simulink model "rob_kuka_sim"  (R2018b)
settings: Solver=VariableStepAuto  StartTime=0.0  StopTime=90  RelTol=1e-3
values from neighbouring files (symbols this model uses):
  L_SB = 14.173    [rob_kuka.m]    (also in rob_kuka_pose.m)
  T = [T; 0,0,0,1]    [forKine.m]    (also in rob_kuka.m = zeros(n*4,4); rob_kuka_pose.m = zeros(n*4,4))
libraries: vrlib x17, dspmtrx3 x4
settings Model: Creator=szhao3  LastModifiedBy=szhao3
settings SFSimCC: SimUseLocalCustomCode=off
settings RTWCC: RTWUseLocalCustomCode=off

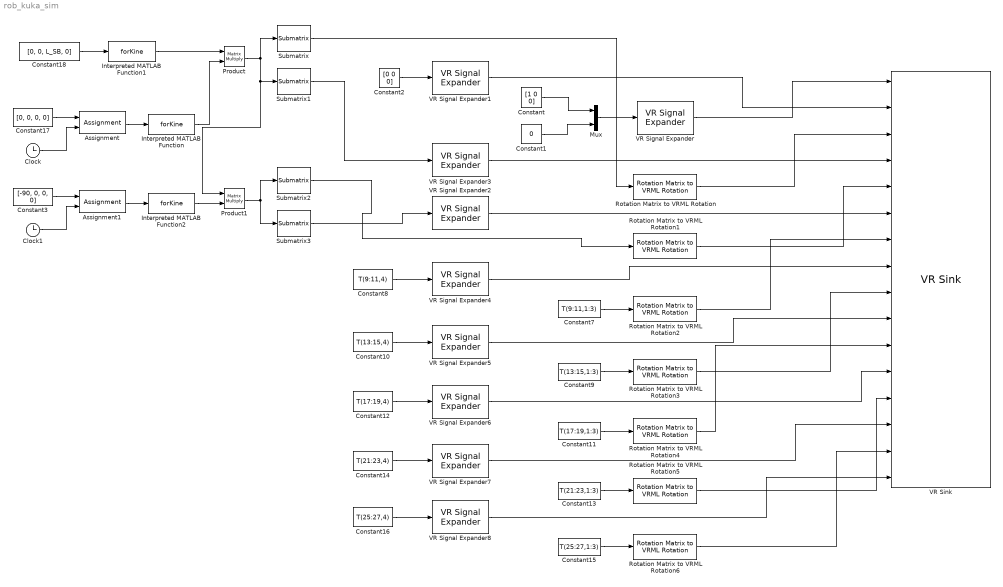
== system rob_kuka_sim ==
  Assignment : Assignment  DiagnosticForDimensions=Warning  IndexOptions=Index vector (dialog)  Indices=4  OutputSizes=1
  Assignment1 : Assignment  DiagnosticForDimensions=Warning  IndexOptions=Index vector (dialog)  Indices=4  OutputSizes=1
  Clock : Clock
  Clock1 : Clock
  Constant : Constant  Value=[1 0 0]  VectorParams1D=off
  Constant1 : Constant  Value=0
  Constant10 : Constant  Value=T(13:15,4)  VectorParams1D=off
  Constant11 : Constant  Value=T(17:19,1:3)  VectorParams1D=off
  Constant12 : Constant  Value=T(17:19,4)  VectorParams1D=off
  Constant13 : Constant  Value=T(21:23,1:3)  VectorParams1D=off
  Constant14 : Constant  Value=T(21:23,4)  VectorParams1D=off
  Constant15 : Constant  Value=T(25:27,1:3)  VectorParams1D=off
  Constant16 : Constant  Value=T(25:27,4)  VectorParams1D=off
  Constant17 : Constant  Value=[0, 0, 0, 0]  VectorParams1D=off
  Constant18 : Constant  Value=[0, 0, L_SB, 0]  VectorParams1D=off
  Constant2 : Constant  Value=[0 0 0]  VectorParams1D=off
  Constant3 : Constant  Value=[-90, 0, 0, 0]  VectorParams1D=off
  Constant7 : Constant  Value=T(9:11,1:3)  VectorParams1D=off
  Constant8 : Constant  Value=T(9:11,4)  VectorParams1D=off
  Constant9 : Constant  Value=T(13:15,1:3)  VectorParams1D=off
  Interpreted MATLAB Function : MATLABFcn  MATLABFcn=forKine  Output1D=off
  Interpreted MATLAB Function1 : MATLABFcn  MATLABFcn=forKine  Output1D=off
  Interpreted MATLAB Function2 : MATLABFcn  MATLABFcn=forKine  Output1D=off
  Mux : Mux  Inputs=2
  Product : Product  Multiplication=Matrix(*)
  Product1 : Product  Multiplication=Matrix(*)
  Rotation Matrix to VRML Rotation{,1..6} (7 alike) : vrlib/Utilities/Rotation Matrix to VRML Rotation  maxzero=1e-12
      settings: SourceProductName=Simulink 3D Animation  SourceProductBaseCode=VR
  Submatrix : dspmtrx3/Submatrix  RowSpan=Range of rows  RowStartMode=First  RowStartIndex=1  RowEndMode=Index  RowEndIndex=3  ColSpan=Range of columns  ColStartMode=First  ColStartIndex=1  ColEndMode=Index  ColEndIndex=3
  Submatrix1 : dspmtrx3/Submatrix  RowSpan=Range of rows  RowStartMode=First  RowStartIndex=1  RowEndMode=Index  RowEndIndex=3  ColSpan=One column  ColStartMode=Last  ColStartIndex=1  ColEndMode=Index  ColEndIndex=3
  Submatrix2 : dspmtrx3/Submatrix  RowSpan=Range of rows  RowStartMode=First  RowStartIndex=1  RowEndMode=Index  RowEndIndex=3  ColSpan=Range of columns  ColStartMode=First  ColStartIndex=1  ColEndMode=Index  ColEndIndex=3
  Submatrix3 : dspmtrx3/Submatrix  RowSpan=Range of rows  RowStartMode=First  RowStartIndex=1  RowEndMode=Index  RowEndIndex=3  ColSpan=One column  ColStartMode=Last  ColStartIndex=1  ColEndMode=Index  ColEndIndex=3
  VR Signal Expander : vrlib/VR Signal Expander  outwidth=4  outidx=[1 2 3 4]
      settings: SourceProductName=Simulink 3D Animation  SourceProductBaseCode=VR
  VR Signal Expander{1..8} (8 alike) : vrlib/VR Signal Expander  outwidth=3  outidx=[1 2 3]
      settings: SourceProductName=Simulink 3D Animation  SourceProductBaseCode=VR
  VR Sink : vrlib/VR Sink  InstantiateOnLoad=on  SampleTime=0.1  ViewEnable=on  RemoteChange=off  RemoteView=off  FieldsWritten=B.rotation.4.1.1.double#B.translation.3.1.1.double#R1.rotation.4.1.1.double#R1.translation.3.1.1.double#R2.rotation.4.1.1.double#R2.translation.3.1.1.double#R3.rotation.4.1.1.double#R3.translation.3.1.1.double#R4.rotation.4.1.1.double#R4.translation.3.1.1.double#R5.rotation.4.1.1.double#R5.translation.3.1.1.double#R6.rotation.4.1.1.double#R6.translation.3.1.1.double#R7.rotation.4.1.1.double#R7.translation.3.1.1.double  WorldFileName=..\WRL2\lbr iiwa 14 r820-wrl.wrl  AutoView=off  VideoDimensions=[]  AllowVariableSize=off
      settings: SourceProductBaseCode=VR
  wires:
  Mux/1 -> VR Signal Expander/1
  Constant/1 -> Mux/1
  Constant1/1 -> Mux/2
  Constant2/1 -> VR Signal Expander1/1
  Submatrix/1 -> Rotation Matrix to VRML Rotation/1
  Submatrix3/1 -> VR Signal Expander2/1
  Submatrix2/1 -> Rotation Matrix to VRML Rotation1/1
  Constant8/1 -> VR Signal Expander4/1
  Constant7/1 -> Rotation Matrix to VRML Rotation2/1
  Constant9/1 -> Rotation Matrix to VRML Rotation3/1
  Constant10/1 -> VR Signal Expander5/1
  Constant11/1 -> Rotation Matrix to VRML Rotation4/1
  Constant12/1 -> VR Signal Expander6/1
  Constant13/1 -> Rotation Matrix to VRML Rotation5/1
  Constant14/1 -> VR Signal Expander7/1
  Constant15/1 -> Rotation Matrix to VRML Rotation6/1
  Constant16/1 -> VR Signal Expander8/1
  Constant17/1 -> Assignment/1
  Assignment/1 -> Interpreted MATLAB Function/1
  Interpreted MATLAB Function/1 -> Product/2
  Constant18/1 -> Interpreted MATLAB Function1/1
  Interpreted MATLAB Function1/1 -> Product/1
  Product/1 -> Submatrix/1, Product1/1, Submatrix1/1
  Submatrix1/1 -> VR Signal Expander3/1
  Clock/1 -> Assignment/2
  Constant3/1 -> Assignment1/1
  Assignment1/1 -> Interpreted MATLAB Function2/1
  Clock1/1 -> Assignment1/2
  Interpreted MATLAB Function2/1 -> Product1/2
  Product1/1 -> Submatrix3/1, Submatrix2/1
  VR Signal Expander/1 -> VR Sink/1
  VR Signal Expander1/1 -> VR Sink/2
  Rotation Matrix to VRML Rotation/1 -> VR Sink/3
  VR Signal Expander3/1 -> VR Sink/4
  Rotation Matrix to VRML Rotation1/1 -> VR Sink/5
  VR Signal Expander2/1 -> VR Sink/6
  Rotation Matrix to VRML Rotation2/1 -> VR Sink/7
  VR Signal Expander4/1 -> VR Sink/8
  Rotation Matrix to VRML Rotation3/1 -> VR Sink/9
  VR Signal Expander5/1 -> VR Sink/10
  Rotation Matrix to VRML Rotation4/1 -> VR Sink/11
  VR Signal Expander6/1 -> VR Sink/12
  Rotation Matrix to VRML Rotation5/1 -> VR Sink/13
  VR Signal Expander7/1 -> VR Sink/14
  Rotation Matrix to VRML Rotation6/1 -> VR Sink/15
  VR Signal Expander8/1 -> VR Sink/16
